simulink model "sim12ex10d"  (Simulink 2.09)
settings: Solver=ode45  StartTime=0.0  StopTime=3  MaxStep=.050  RelTol=1e-3  AbsTol=1e-3
settings Model: SaveTime=off  SaveOutput=off  ConsistencyChecking=off  RTWTemplateMakefile=grt_vc.tmf

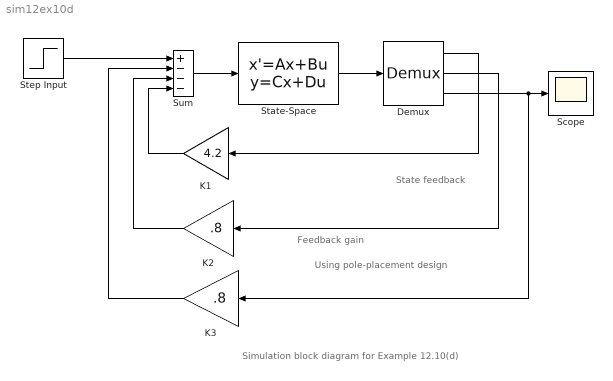
== system sim12ex10d ==
  note: Simulation block diagram for Example 12.10(d)
  note: Using pole-placement design
  note: Feedback gain
  note: State feedback
  Demux : Demux  Outputs=3
  K1 : Gain  Orientation=left  Gain=4.2
  K2 : Gain  Orientation=left  Gain=.8
  K3 : Gain  Orientation=left  Gain=.8
  Scope : Scope
      settings: TickLabels=on  TimeRange=auto  YMin=-5  YMax=5  SaveToWorkspace=off  SaveName=ScopeData
  State-Space : StateSpace  A="[-5  0  -100;  2  -2  0;  0  0.1  -0.08]"  B="[0;   0 ;  -0.1]"  C=eye(3)  D=zeros(3, 1)  X0=0
  Step Input : Step  Time=10  Before=0.2  After=.2
  Sum : Sum  Inputs=+---
  wires:
  K3/1 -> Sum/2
  Demux/3 -> K3/1, Scope/1
  Step Input/1 -> Sum/1
  K2/1 -> Sum/3
  K1/1 -> Sum/4
  Sum/1 -> State-Space/1
  Demux/2 -> K2/1
  Demux/1 -> K1/1
  State-Space/1 -> Demux/1
